simulink model "MsgEthernetMdl"  (R2022a)
settings: Solver=VariableStepAuto  StartTime=0.0  StopTime=30  FixedStep=1  MaxStep=Inf  RelTol=1e-3  EnableMultiTasking=on
PreLoadFcn:
  | load ethernetTypes.mat;
InitFcn:
  | BitRate = 10e6;
values from neighbouring files (symbols this model uses):
  n = length(stations)    [ethernetHubMask.m]
undefined symbols (not defined in the file or in its folder): gateControl, m, networkselector
libraries: matrix_library x4
(part 1 of 2)
settings Model: Creator=The MathWorks, Inc.  LastModifiedBy=lch
settings SolverCC: AlgebraicLoopSolver=TrustRegion
settings DataIOCC: ReturnWorkspaceOutputs=off
settings OptimizationCC: LifeSpan=inf
settings DebuggingCC: UnconnectedInputMsg=warning  UnconnectedOutputMsg=warning  UnconnectedLineMsg=warning  SFUnexpectedBacktrackingDiag=warning  SFNoUnconditionalDefaultTransitionDiag=warning  SFMachineParentedDataDiag=warning  ArithmeticOperatorsInVariantConditions=warning
settings SFSimCC: SimUseLocalCustomCode=off  CustomCodeUndefinedFunction=UseInterfaceOnly
settings RTWCC: RTWUseLocalCustomCode=off
settings CodeAppCC: StateflowObjectComments=on
settings GRTTargetCC: TargetLangStandard=C89/C90 (ANSI)
settings ConfigComp: CovMetricSettings=dw  CovSaveCumulativeToWorkspaceVar=on  CovSaveSingleToWorkspaceVar=on  CovExternalEMLEnable=off

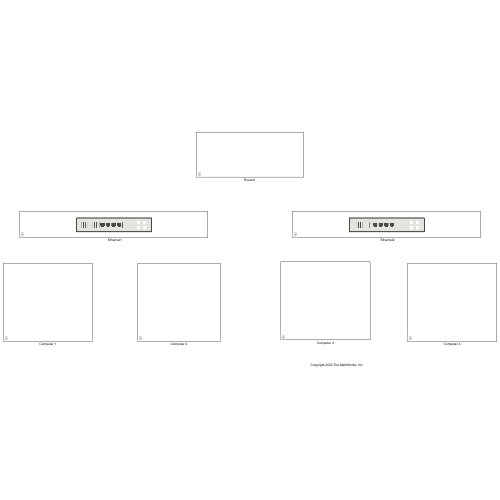
[thumbnail: Simulink's stored preview of the top-level diagram]
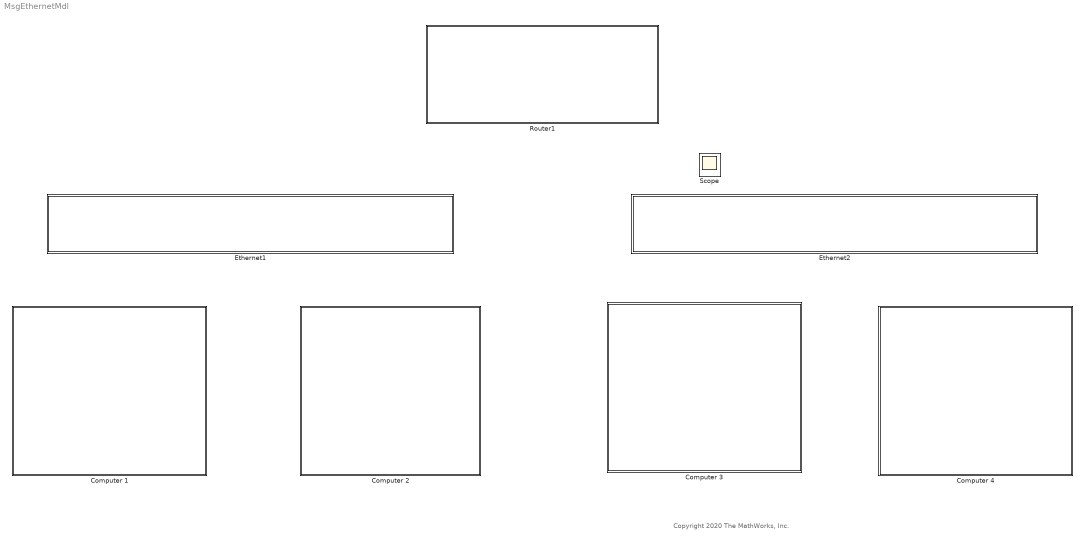
== system MsgEthernetMdl ==
  note: Copyright 2020 The MathWorks, Inc.
  "   Ethernet1" : Subsystem  mask(Ethernet Hub){Stations=[2 1], CableLength=[300 100], PER=[0 0], ProcessingTime=0, ip=[10 1 1 1]}
      mask prompts: Stations "Connected stations"; CableLength "Length of cables (m)"; PER "Packet error rate (PER)"; ProcessingTime "Processing time (s)"
      mask help: Connect Ethernet stations
      mask init:
      | if length(Stations) < 2
      |     error('Number of connected stations must be greater than 1');
      | end
      | if length(CableLength) ~= length(Stations)
      |     error('Parameter ''Length of cables'' must be a vector with number of elements equals to number of connected stations');
      | end
      | if length(PER) ~= length(Stations)
      |     error('Parameter ''Packet error rate'' must be a vector with number of elements equals to number of connected stations');
      | end
      mask DialogControl Container2 Prompt: Parameters
      mask Display: image('ethernet-illustration.png')
  "   Ethernet2" : Subsystem  mask(Ethernet Hub){Stations=[3 2 1], CableLength=[200 300 100], PER=[0 0 0], ProcessingTime=0, ip=[10 1 2 1]}
      mask prompts: Stations "Connected stations"; CableLength "Length of cables (m)"; PER "Packet error rate (PER)"; ProcessingTime "Processing time (s)"
      mask help: Connect Ethernet stations
      mask init: same as MsgEthernetMdl/   Ethernet1
      mask DialogControl Container2 Prompt: Parameters
      mask Display: image('ethernet-illustration.png')
  Computer 1 : Subsystem  mask{ip=[10 1 1 2], netmask=[255 255 255 0], gateway=[10 1 1 1]}
      mask prompts: ip "IP Address"
      mask DialogControl ParameterGroupVar Prompt: 파라미터
  Computer 2 : Subsystem  mask{ip=[10 1 1 3], netmask=[255 255 255 0], gateway=[10 1 1 1]}
      mask prompts: ip "IP Address"
      mask DialogControl ParameterGroupVar Prompt: 파라미터
  Computer 3 : Subsystem  mask{ip=[10 1 2 2], netmask=[255 255 255 0], gateway=[10 1 2 1]}
      mask prompts: ip "IP Address"
      mask DialogControl ParameterGroupVar Prompt: 파라미터
  Computer 4 : Subsystem  mask{ip=[10 1 2 3], netmask=[255 255 255 0], gateway=[10 1 2 1]}
      mask prompts: ip "IP Address"
      mask DialogControl ParameterGroupVar Prompt: 파라미터
  Router1 : Subsystem  mask{vlan1=[10 1 1], vlan2=[10 1 2]}
      mask DialogControl ParameterGroupVar Prompt: 파라미터
  Scope : Scope

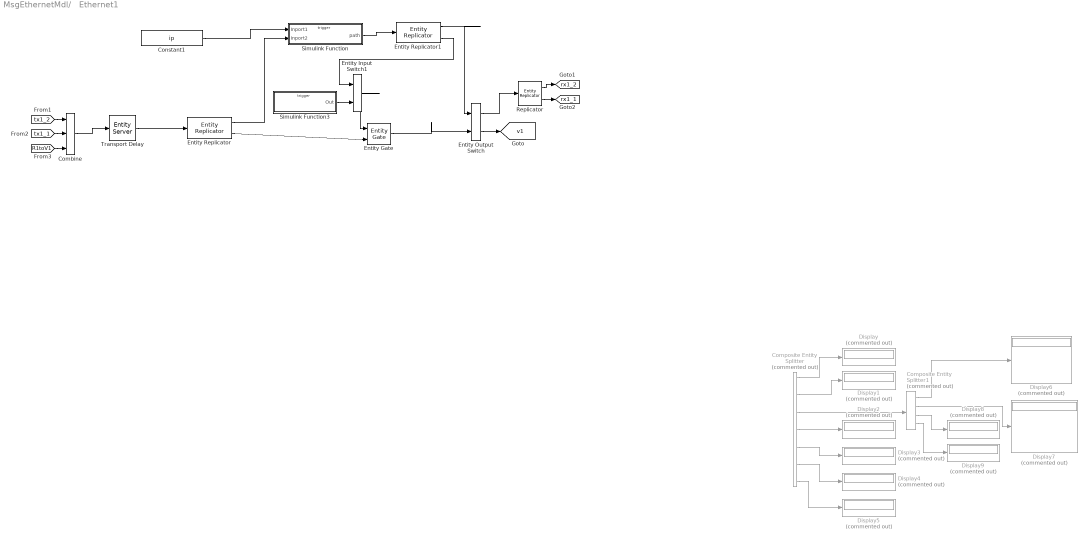
== system MsgEthernetMdl/   Ethernet1 ==
  Combine : EntityInputSwitch  InputPortMessageModes=m,m,m  OutputPortMessageModes=m  NumberInputPorts=3
      settings: InputPortMap=u1,u2,u3
  Composite Entity Splitter : CompositeEntitySplitter  Commented=on  InputPortMessageModes=m  OutputPortMessageModes=m,m,m,m,m,m,m  NumberOutputPorts=7
      settings: OutputPortMap=o0,o1,o2,o3,o4,o5,o6
  Composite Entity Splitter1 : CompositeEntitySplitter  Commented=on  InputPortMessageModes=m  OutputPortMessageModes=m,m,m,m  NumberOutputPorts=4
      settings: OutputPortMap=o0,o1,o2,o3
  Constant1 : Constant  Value=ip
  Display{,1..9} (10 alike) : Display  Commented=on
  Entity Input Switch1 : EntityInputSwitch  InputPortMessageModes=m,m  OutputPortMessageModes=m
  Entity Output Switch : EntityOutputSwitch  InputPortMessageModes=m,m  OutputPortMessageModes=m,m  SwitchingCriterion=From control port  SwitchAttributeName=Attribute1
      settings: InputPortMap=u0,u1
  Entity Gate : EntityGate  InputPortMessageModes=m,m  OutputPortMessageModes=m  OpenGateAtSimulationStart=on
  Entity Replicator : EntityReplicator  InputPortMessageModes=m  OutputPortMessageModes=m,m
  Entity Replicator1 : EntityReplicator  InputPortMessageModes=m  OutputPortMessageModes=m,m
  Replicator : EntityReplicator  InputPortMessageModes=m  OutputPortMessageModes=m,m
  Simulink Function : Subsystem  TreatAsAtomicUnit=on
  Simulink Function3 : Subsystem  TreatAsAtomicUnit=on
  Transport Delay : EntityServer  InputPortMessageModes=m  OutputPortMessageModes=m  Capacity=Inf  ServiceTimeSource=MATLAB action  ServiceTimeAction=|  ServiceCompleteAction=|  ExitAction=gateControl();
      ServiceTimeAction=|
      | src = entity.TxAddress;
      | dst = entity.RxAddress;
      | srcl = 0;
      | dstl = 0;
      | for i = 1:length(Stations)
      |     if src == Stations(i)
      |         srcl = CableLength(i);
      |     end
      |     if dst == Stations(i)
      |         dstl = CableLength(i);
      |     end
      |     if srcl > 0 && dstl > 0
      |         break;
      |     end
      | end
      | dt = ProcessingTime + (srcl + dstl)/3e8;
      ServiceCompleteAction=|
      | networkselector();
      | src = entity.TxAddress;
      | dst = entity.RxAddress;
      | srcIdx = 0;
      | dstIdx = 0;
      | for i = 1:length(Stations)
      |     if src == Stations(i)
      |         srcIdx = i;
      |     end
      |     if dst == Stations(i)
      |         dstIdx = i;
      |     end
      |     if srcIdx > 0 && dstIdx > 0
      |         break;
      |     end
      | end
      | if rand < (PER(srcIdx) + PER(dstIdx))
      |     entity.CRC = 1;
      | end
  tag scope: rx1_1=global, rx1_2=global, v1=global
  wires:
  Combine/1 -> Transport Delay/1
  Transport Delay/1 -> Entity Replicator/1
  [tx1_2] -> Combine/1
  Replicator/1 -> [rx1_2]
  [tx1_1] -> Combine/2
  Replicator/2 -> [rx1_1]
  Entity Output Switch/1 -> Replicator/1
  [R1toV1] -> Combine/3
  Entity Gate/1 -> Entity Output Switch/2
  Simulink Function/1(path) -> Entity Replicator1/1
  Simulink Function3/1(Out) -> Entity Input Switch1/2
  Entity Input Switch1/1 -> Entity Gate/1
  Entity Replicator1/2 -> Entity Input Switch1/1
  Entity Replicator1/1 -> Entity Output Switch/1
  Entity Replicator/2 -> Entity Gate/2
  Entity Replicator/1 -> Simulink Function/2(Inport2)
  Constant1/1 -> Simulink Function/1(Inport1)
  Composite Entity Splitter/2 -> Display1/1
  Composite Entity Splitter1/4 -> Display9/1
  Composite Entity Splitter1/3 -> Display8/1
  Composite Entity Splitter/5 -> Display3/1
  Composite Entity Splitter/4 -> Display2/1
  Composite Entity Splitter/1 -> Display/1
  Composite Entity Splitter/7 -> Display5/1
  Composite Entity Splitter/6 -> Display4/1
  Composite Entity Splitter1/2 -> Display7/1
  Composite Entity Splitter/3 -> Composite Entity Splitter1/1
  Composite Entity Splitter1/1 -> Display6/1
  Entity Output Switch/2 -> [v1]

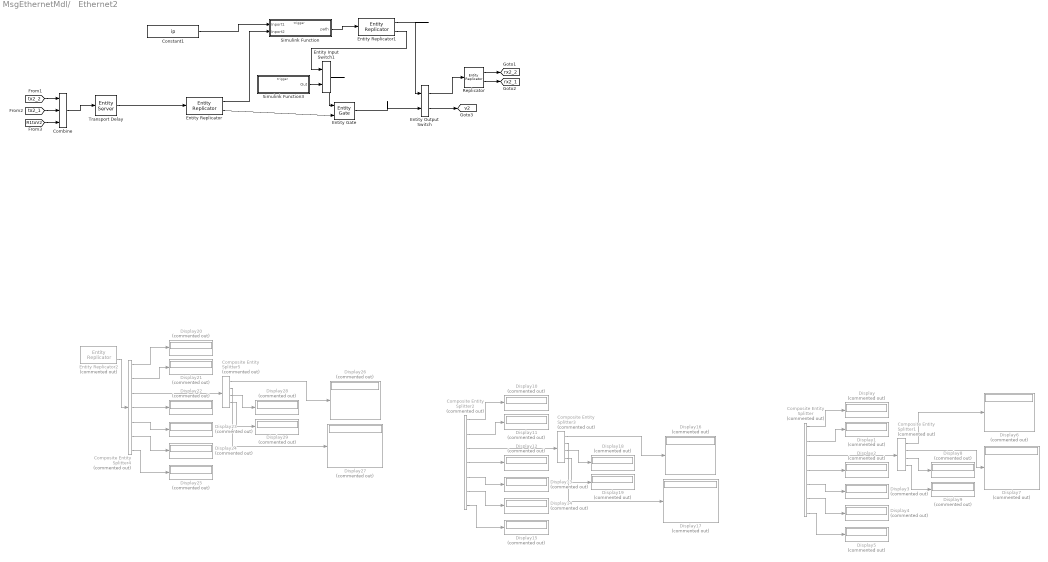
== system MsgEthernetMdl/   Ethernet2 ==
  Combine : EntityInputSwitch  InputPortMessageModes=m,m,m  OutputPortMessageModes=m  NumberInputPorts=3
      settings: InputPortMap=u1,u2,u3
  Composite Entity Splitter : CompositeEntitySplitter  Commented=on  InputPortMessageModes=m  OutputPortMessageModes=m,m,m,m,m,m,m  NumberOutputPorts=7
      settings: OutputPortMap=o0,o1,o2,o3,o4,o5,o6
  Composite Entity Splitter1 : CompositeEntitySplitter  Commented=on  InputPortMessageModes=m  OutputPortMessageModes=m,m,m,m  NumberOutputPorts=4
      settings: OutputPortMap=o0,o1,o2,o3
  Composite Entity Splitter2 : CompositeEntitySplitter  Commented=on  InputPortMessageModes=m  OutputPortMessageModes=m,m,m,m,m,m,m  NumberOutputPorts=7
      settings: OutputPortMap=o0,o1,o2,o3,o4,o5,o6
  Composite Entity Splitter3 : CompositeEntitySplitter  Commented=on  InputPortMessageModes=m  OutputPortMessageModes=m,m,m,m  NumberOutputPorts=4
      settings: OutputPortMap=o0,o1,o2,o3
  Composite Entity Splitter4 : CompositeEntitySplitter  Commented=on  InputPortMessageModes=m  OutputPortMessageModes=m,m,m,m,m,m,m  NumberOutputPorts=7
      settings: OutputPortMap=o0,o1,o2,o3,o4,o5,o6
  Composite Entity Splitter5 : CompositeEntitySplitter  Commented=on  InputPortMessageModes=m  OutputPortMessageModes=m,m,m,m  NumberOutputPorts=4
      settings: OutputPortMap=o0,o1,o2,o3
  Constant1 : Constant  Value=ip
  Display{,1..29} (30 alike) : Display  Commented=on
  Entity Input Switch1 : EntityInputSwitch  InputPortMessageModes=m,m  OutputPortMessageModes=m
  Entity Output Switch : EntityOutputSwitch  InputPortMessageModes=m,m  OutputPortMessageModes=m,m  SwitchingCriterion=From control port  SwitchAttributeName=Attribute1
      settings: InputPortMap=u0,u1
  Entity Gate : EntityGate  InputPortMessageModes=m,m  OutputPortMessageModes=m  OpenGateAtSimulationStart=on
  Entity Replicator : EntityReplicator  InputPortMessageModes=m  OutputPortMessageModes=m,m
  Entity Replicator1 : EntityReplicator  InputPortMessageModes=m  OutputPortMessageModes=m,m
  Entity Replicator2 : EntityReplicator  Commented=on  InputPortMessageModes=m  OutputPortMessageModes=m,m
  Replicator : EntityReplicator  InputPortMessageModes=m  OutputPortMessageModes=m,m
  Simulink Function : Subsystem  TreatAsAtomicUnit=on
  Simulink Function3 : Subsystem  TreatAsAtomicUnit=on
  Transport Delay : EntityServer  InputPortMessageModes=m  OutputPortMessageModes=m  Capacity=Inf  ServiceTimeSource=MATLAB action  ServiceTimeAction=|  ServiceCompleteAction=|  ExitAction=gateControl();
      ServiceTimeAction=|
      | src = entity.TxAddress;
      | dst = entity.RxAddress;
      | srcl = 0;
      | dstl = 0;
      | for i = 1:length(Stations)
      |     if src == Stations(i)
      |         srcl = CableLength(i);
      |     end
      |     if dst == Stations(i)
      |         dstl = CableLength(i);
      |     end
      |     if srcl > 0 && dstl > 0
      |         break;
      |     end
      | end
      | dt = ProcessingTime + (srcl + dstl)/3e8;
      ServiceCompleteAction=|
      | networkselector();
      | src = entity.TxAddress;
      | dst = entity.RxAddress;
      | srcIdx = 0;
      | dstIdx = 0;
      | for i = 1:length(Stations)
      |     if src == Stations(i)
      |         srcIdx = i;
      |     end
      |     if dst == Stations(i)
      |         dstIdx = i;
      |     end
      |     if srcIdx > 0 && dstIdx > 0
      |         break;
      |     end
      | end
      | if rand < (PER(srcIdx) + PER(dstIdx))
      |     entity.CRC = 1;
      | end
  tag scope: rx2_1=global, rx2_2=global, v2=global
  wires:
  Combine/1 -> Transport Delay/1
  Entity Output Switch/1 -> Replicator/1
  [tx2_2] -> Combine/1
  Replicator/1 -> [rx2_2]
  [tx2_1] -> Combine/2
  Replicator/2 -> [rx2_1]
  [R1toV2] -> Combine/3
  Composite Entity Splitter1/2 -> Display7/1
  Composite Entity Splitter1/4 -> Display9/1
  Composite Entity Splitter/7 -> Display5/1
  Composite Entity Splitter/1 -> Display/1
  Composite Entity Splitter/2 -> Display1/1
  Composite Entity Splitter/6 -> Display4/1
  Composite Entity Splitter/4 -> Display2/1
  Composite Entity Splitter1/3 -> Display8/1
  Composite Entity Splitter/3 -> Composite Entity Splitter1/1
  Composite Entity Splitter1/1 -> Display6/1
  Composite Entity Splitter/5 -> Display3/1
  Composite Entity Splitter2/5 -> Display13/1
  Composite Entity Splitter3/1 -> Display16/1
  Composite Entity Splitter2/3 -> Composite Entity Splitter3/1
  Composite Entity Splitter3/3 -> Display18/1
  Composite Entity Splitter2/4 -> Display12/1
  Composite Entity Splitter2/6 -> Display14/1
  Composite Entity Splitter2/2 -> Display11/1
  Composite Entity Splitter2/1 -> Display10/1
  Composite Entity Splitter2/7 -> Display15/1
  Composite Entity Splitter3/4 -> Display19/1
  Composite Entity Splitter3/2 -> Display17/1
  Entity Replicator/1 -> Simulink Function/2(Inport2)
  Constant1/1 -> Simulink Function/1(Inport1)
  Entity Replicator1/1 -> Entity Output Switch/1
  Entity Replicator1/2 -> Entity Input Switch1/1
  Entity Input Switch1/1 -> Entity Gate/1
  Simulink Function/1(path) -> Entity Replicator1/1
  Simulink Function3/1(Out) -> Entity Input Switch1/2
  Entity Gate/1 -> Entity Output Switch/2
  Entity Replicator/2 -> Entity Gate/2
  Transport Delay/1 -> Entity Replicator/1
  Composite Entity Splitter5/1 -> Display26/1
  Composite Entity Splitter4/7 -> Display25/1
  Composite Entity Splitter4/5 -> Display23/1
  Composite Entity Splitter5/2 -> Display27/1
  Composite Entity Splitter4/6 -> Display24/1
  Composite Entity Splitter4/2 -> Display21/1
  Composite Entity Splitter5/3 -> Display28/1
  Composite Entity Splitter4/1 -> Display20/1
  Composite Entity Splitter5/4 -> Display29/1
  Composite Entity Splitter4/3 -> Composite Entity Splitter5/1
  Composite Entity Splitter4/4 -> Display22/1
  Entity Replicator2/2 -> Composite Entity Splitter4/1
  Entity Output Switch/2 -> [v2]

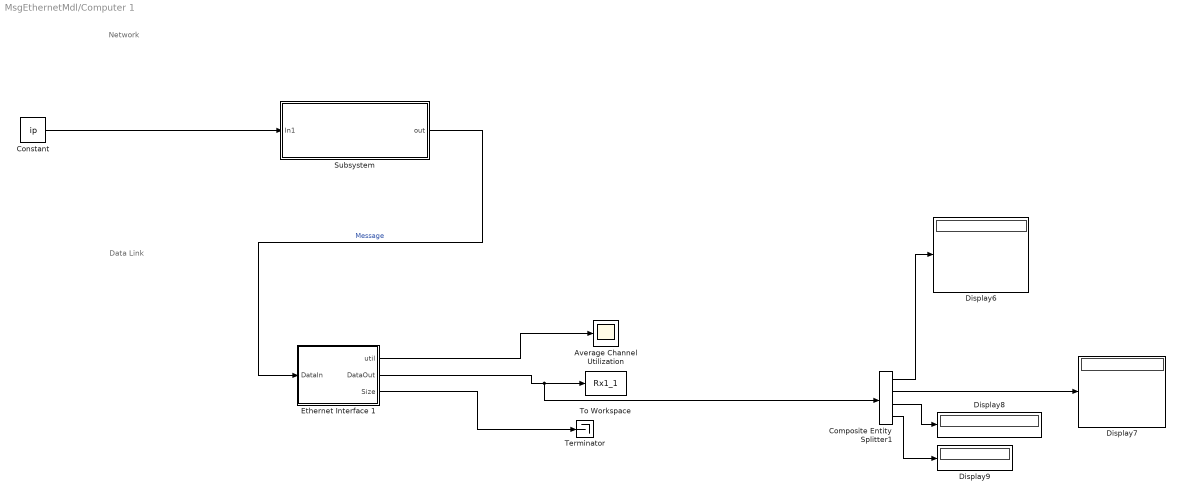
== system MsgEthernetMdl/Computer 1 ==
  note: Network
  note: Data Link
  Average Channel Utilization : Scope
  Composite Entity Splitter1 : CompositeEntitySplitter  InputPortMessageModes=m  OutputPortMessageModes=m,m,m,m  NumberOutputPorts=4
      settings: OutputPortMap=o0,o1,o2,o3
  Constant : Constant  Value=ip
  Display{6..9} (4 alike) : Display
  Ethernet Interface 1 : Subsystem  mask(Ethernet MAC Layer){StationID=1, TxBufferCapacity=256}
      mask prompts: StationID "Station ID"; TxBufferCapacity "Transmission buffer capacity"
      mask help: Ethernet MAC layer packet transmission and reception based on CSMA/CD
      mask Display: image('ethernet-interface-illustration.png')
  Subsystem : Subsystem
  Terminator : Terminator
  To Workspace : ToWorkspace  VariableName=Rx1_1  SaveFormat=Timeseries  SampleTime=-1
  wires:
  Ethernet Interface 1/3(Size) -> Terminator/1
  Subsystem/1(out) -> Ethernet Interface 1/1(DataIn)  "Message"
  Ethernet Interface 1/1(util) -> Average Channel Utilization/1
  Constant/1 -> Subsystem/1(In1)
  Composite Entity Splitter1/1 -> Display6/1
  Composite Entity Splitter1/3 -> Display8/1
  Composite Entity Splitter1/4 -> Display9/1
  Composite Entity Splitter1/2 -> Display7/1
  Ethernet Interface 1/2(DataOut) -> Composite Entity Splitter1/1, To Workspace/1

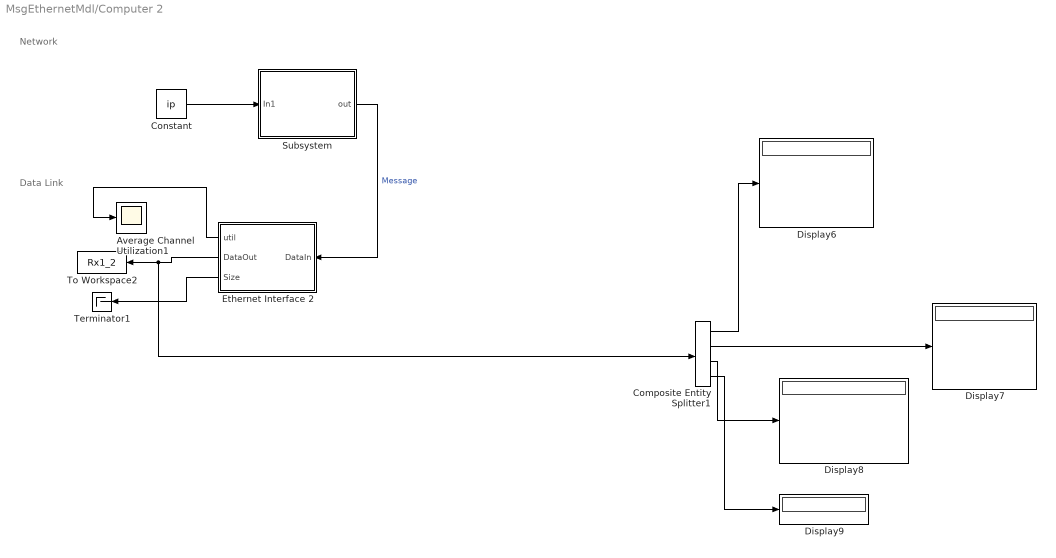
== system MsgEthernetMdl/Computer 2 ==
  note: Network
  note: Data Link
  Average Channel Utilization1 : Scope
  Composite Entity Splitter1 : CompositeEntitySplitter  InputPortMessageModes=m  OutputPortMessageModes=m,m,m,m  NumberOutputPorts=4
      settings: OutputPortMap=o0,o1,o2,o3
  Constant : Constant  Value=ip
  Display{6..9} (4 alike) : Display
  Ethernet Interface 2 : Subsystem  mask(Ethernet MAC Layer){StationID=2, TxBufferCapacity=256}
      mask prompts: StationID "Station ID"; TxBufferCapacity "Transmission buffer capacity"
      mask help: Ethernet MAC layer packet transmission and reception based on CSMA/CD
      mask Display: image('ethernet-interface-illustration.png')
  Subsystem : Subsystem
  Terminator1 : Terminator
  To Workspace2 : ToWorkspace  VariableName=Rx1_2  SaveFormat=Timeseries  SampleTime=-1
  wires:
  Ethernet Interface 2/3(Size) -> Terminator1/1
  Subsystem/1(out) -> Ethernet Interface 2/1(DataIn)  "Message"
  Ethernet Interface 2/1(util) -> Average Channel Utilization1/1
  Constant/1 -> Subsystem/1(In1)
  Composite Entity Splitter1/3 -> Display8/1
  Composite Entity Splitter1/2 -> Display7/1
  Composite Entity Splitter1/4 -> Display9/1
  Composite Entity Splitter1/1 -> Display6/1
  Ethernet Interface 2/2(DataOut) -> Composite Entity Splitter1/1, To Workspace2/1

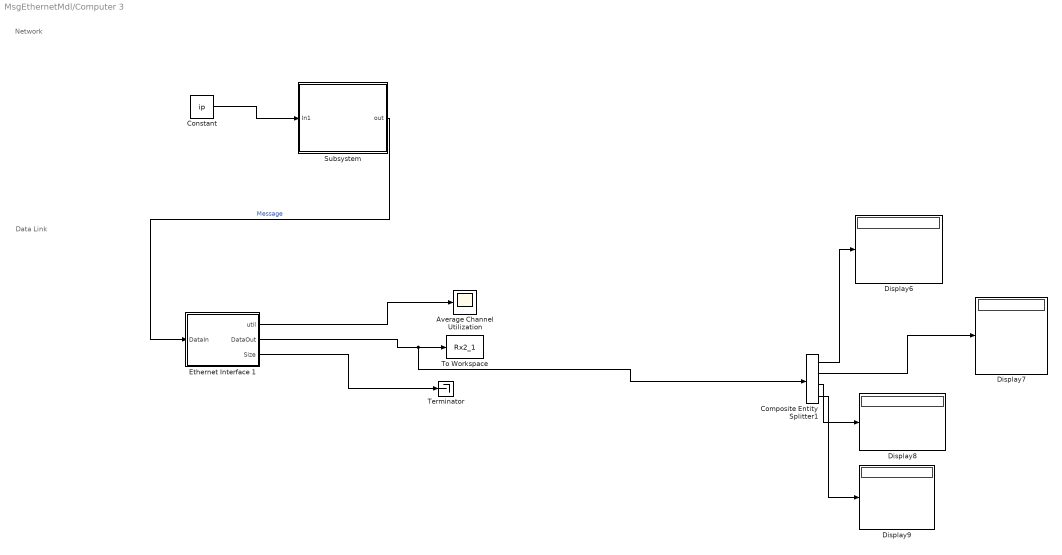
== system MsgEthernetMdl/Computer 3 ==
  note: Network
  note: Data Link
  Average Channel Utilization : Scope
  Composite Entity Splitter1 : CompositeEntitySplitter  InputPortMessageModes=m  OutputPortMessageModes=m,m,m,m  NumberOutputPorts=4
      settings: OutputPortMap=o0,o1,o2,o3
  Constant : Constant  Value=ip
  Display{6..9} (4 alike) : Display
  Ethernet Interface 1 : Subsystem  mask(Ethernet MAC Layer){StationID=1, TxBufferCapacity=256}
      mask prompts: StationID "Station ID"; TxBufferCapacity "Transmission buffer capacity"
      mask help: Ethernet MAC layer packet transmission and reception based on CSMA/CD
      mask Display: image('ethernet-interface-illustration.png')
  Subsystem : Subsystem
  Terminator : Terminator
  To Workspace : ToWorkspace  VariableName=Rx2_1  SaveFormat=Timeseries  SampleTime=-1
  wires:
  Ethernet Interface 1/3(Size) -> Terminator/1
  Subsystem/1(out) -> Ethernet Interface 1/1(DataIn)  "Message"
  Ethernet Interface 1/1(util) -> Average Channel Utilization/1
  Constant/1 -> Subsystem/1(In1)
  Ethernet Interface 1/2(DataOut) -> Composite Entity Splitter1/1, To Workspace/1
  Composite Entity Splitter1/3 -> Display8/1
  Composite Entity Splitter1/2 -> Display7/1
  Composite Entity Splitter1/4 -> Display9/1
  Composite Entity Splitter1/1 -> Display6/1

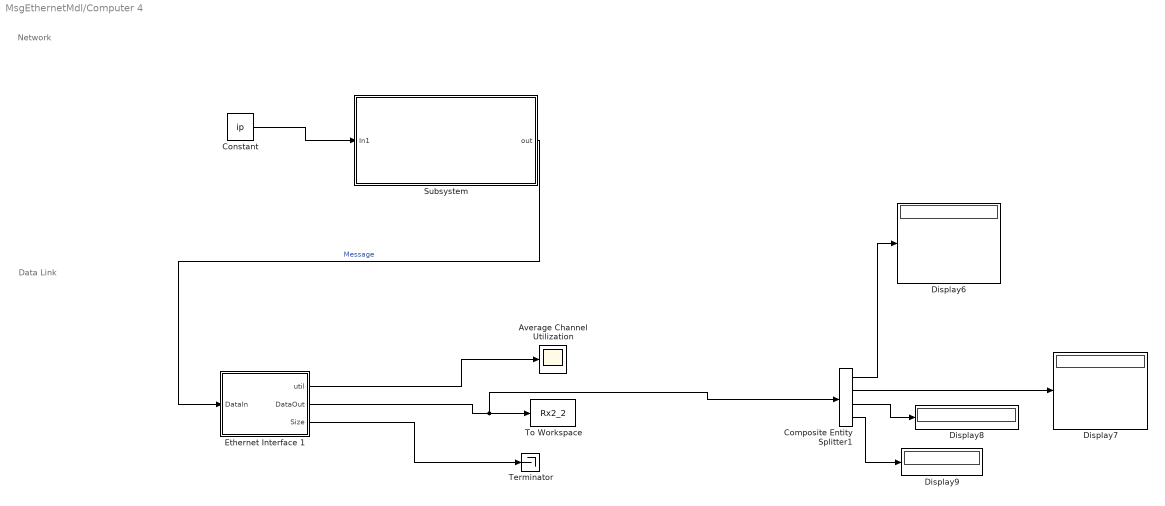
== system MsgEthernetMdl/Computer 4 ==
  note: Network
  note: Data Link
  Average Channel Utilization : Scope
  Composite Entity Splitter1 : CompositeEntitySplitter  InputPortMessageModes=m  OutputPortMessageModes=m,m,m,m  NumberOutputPorts=4
      settings: OutputPortMap=o0,o1,o2,o3
  Constant : Constant  Value=ip
  Display{6..9} (4 alike) : Display
  Ethernet Interface 1 : Subsystem  mask(Ethernet MAC Layer){StationID=2, TxBufferCapacity=256}
      mask prompts: StationID "Station ID"; TxBufferCapacity "Transmission buffer capacity"
      mask help: Ethernet MAC layer packet transmission and reception based on CSMA/CD
      mask Display: image('ethernet-interface-illustration.png')
  Subsystem : Subsystem
  Terminator : Terminator
  To Workspace : ToWorkspace  VariableName=Rx2_2  SaveFormat=Timeseries  SampleTime=-1
  wires:
  Ethernet Interface 1/3(Size) -> Terminator/1
  Subsystem/1(out) -> Ethernet Interface 1/1(DataIn)  "Message"
  Ethernet Interface 1/1(util) -> Average Channel Utilization/1
  Constant/1 -> Subsystem/1(In1)
  Composite Entity Splitter1/3 -> Display8/1
  Composite Entity Splitter1/1 -> Display6/1
  Composite Entity Splitter1/4 -> Display9/1
  Composite Entity Splitter1/2 -> Display7/1
  Ethernet Interface 1/2(DataOut) -> Composite Entity Splitter1/1, To Workspace/1

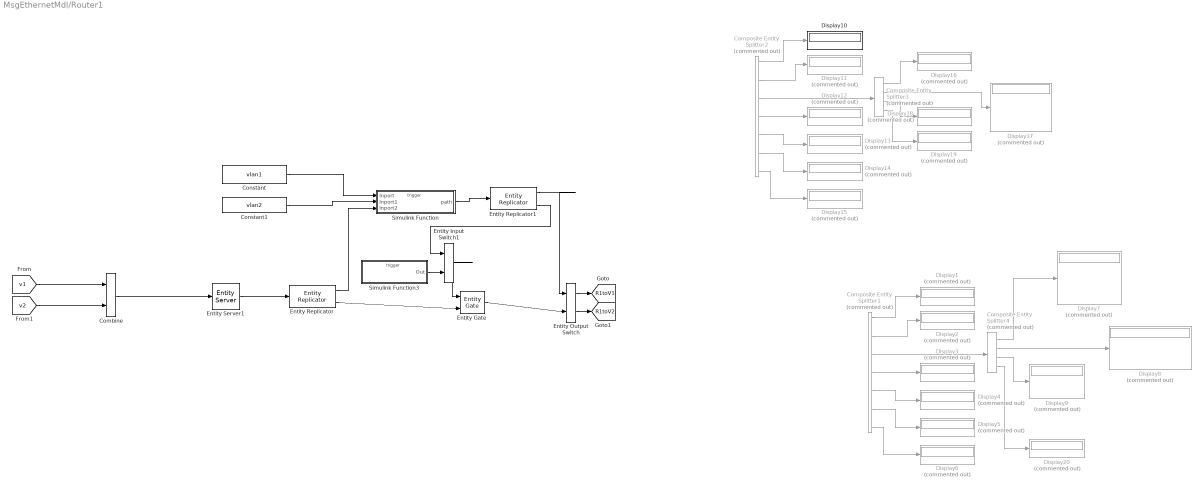
== system MsgEthernetMdl/Router1 ==
  Combine : EntityInputSwitch  InputPortMessageModes=m,m  OutputPortMessageModes=m
  Composite Entity Splitter1 : CompositeEntitySplitter  Commented=on  InputPortMessageModes=m  OutputPortMessageModes=m,m,m,m,m,m,m  NumberOutputPorts=7
      settings: OutputPortMap=o0,o1,o2,o3,o4,o5,o6
  Composite Entity Splitter2 : CompositeEntitySplitter  Commented=on  InputPortMessageModes=m  OutputPortMessageModes=m,m,m,m,m,m,m  NumberOutputPorts=7
      settings: OutputPortMap=o0,o1,o2,o3,o4,o5,o6
  Composite Entity Splitter3 : CompositeEntitySplitter  Commented=on  InputPortMessageModes=m  OutputPortMessageModes=m,m,m,m  NumberOutputPorts=4
      settings: OutputPortMap=o0,o1,o2,o3
  Composite Entity Splitter4 : CompositeEntitySplitter  Commented=on  InputPortMessageModes=m  OutputPortMessageModes=m,m,m,m  NumberOutputPorts=4
      settings: OutputPortMap=o0,o1,o2,o3
  Constant : Constant  Value=vlan1
  Constant1 : Constant  Value=vlan2
  Display{1..9,11..20} (19 alike) : Display  Commented=on
  Display10 : Display
  Entity Input Switch1 : EntityInputSwitch  InputPortMessageModes=m,m  OutputPortMessageModes=m
  Entity Output Switch : EntityOutputSwitch  InputPortMessageModes=m,m  OutputPortMessageModes=m,m  SwitchingCriterion=From control port  SwitchAttributeName=Attribute1
      settings: InputPortMap=u0,u1
  Entity Gate : EntityGate  InputPortMessageModes=m,m  OutputPortMessageModes=m  OpenGateAtSimulationStart=on
  Entity Replicator : EntityReplicator  InputPortMessageModes=m  OutputPortMessageModes=m,m
  Entity Replicator1 : EntityReplicator  InputPortMessageModes=m  OutputPortMessageModes=m,m
  Entity Server1 : EntityServer  InputPortMessageModes=m  OutputPortMessageModes=m  Capacity=inf  ServiceTimeSource=MATLAB action  ServiceCompleteAction=networkselector();  ExitAction=gateControl();
  Simulink Function : Subsystem  TreatAsAtomicUnit=on
  Simulink Function3 : Subsystem  TreatAsAtomicUnit=on
  tag scope: R1toV1=global, R1toV2=global
  wires:
  [v1] -> Combine/1
  Composite Entity Splitter3/4 -> Display19/1
  Composite Entity Splitter2/3 -> Composite Entity Splitter3/1
  Composite Entity Splitter2/5 -> Display13/1
  Composite Entity Splitter2/6 -> Display14/1
  Composite Entity Splitter2/2 -> Display11/1
  Composite Entity Splitter2/7 -> Display15/1
  Composite Entity Splitter3/1 -> Display16/1
  Composite Entity Splitter3/2 -> Display17/1
  Composite Entity Splitter3/3 -> Display18/1
  Composite Entity Splitter2/1 -> Display10/1
  Composite Entity Splitter2/4 -> Display12/1
  Composite Entity Splitter1/1 -> Display1/1
  Composite Entity Splitter4/3 -> Display9/1
  Composite Entity Splitter4/1 -> Display7/1
  Composite Entity Splitter1/5 -> Display4/1
  Composite Entity Splitter1/3 -> Composite Entity Splitter4/1
  Composite Entity Splitter1/4 -> Display3/1
  Composite Entity Splitter4/2 -> Display8/1
  Composite Entity Splitter1/7 -> Display6/1
  Composite Entity Splitter1/2 -> Display2/1
  Composite Entity Splitter4/4 -> Display20/1
  Composite Entity Splitter1/6 -> Display5/1
  [v2] -> Combine/2
  Combine/1 -> Entity Server1/1
  Entity Replicator/2 -> Entity Gate/2
  Entity Gate/1 -> Entity Output Switch/2
  Simulink Function/1(path) -> Entity Replicator1/1
  Entity Input Switch1/1 -> Entity Gate/1
  Simulink Function3/1(Out) -> Entity Input Switch1/2
  Entity Replicator1/2 -> Entity Input Switch1/1
  Entity Replicator1/1 -> Entity Output Switch/1
  Constant1/1 -> Simulink Function/2(Inport1)
  Constant/1 -> Simulink Function/1(Inport)
  Entity Server1/1 -> Entity Replicator/1
  Entity Replicator/1 -> Simulink Function/3(Inport2)
  Entity Output Switch/2 -> [R1toV2]
  Entity Output Switch/1 -> [R1toV1]

== system MsgEthernetMdl/   Ethernet1/Simulink Function ==
  Inport1 : Inport
  Inport2 : Inport  Port=2
  networkselector : TriggerPort  TriggerType=function-call  IsSimulinkFunction=on  FunctionName=networkselector  FunctionVisibility=scoped  VariantControl=(inherit)
  Bus Selector : BusSelector  OutputSignals=Data
  Bus Selector1 : BusSelector  OutputSignals=DestAddress
  Display : Display
  MATLAB Function : MATLAB Function  TreatAsAtomicUnit=on
  Message Send : Send  OutputPortMessageModes=m
  Receive : Receive  InputPortMessageModes=m  UseInternalQueue=off  QueueOverwriting=on  QueueLength=1  QueueType=LIFO
  path : Outport
  wires:
  Receive/1 -> Bus Selector/1
  Inport1/1 -> MATLAB Function/1(v1)
  Bus Selector/1 -> Bus Selector1/1  "<Data>"
  MATLAB Function/1(idx) -> Display/1, Message Send/1
  Message Send/1 -> path/1
  Inport2/1 -> Receive/1
  Bus Selector1/1 -> MATLAB Function/2(dest)  "<DestAddress>"

== system MsgEthernetMdl/   Ethernet1/Simulink Function3 ==
  gateControl : TriggerPort  TriggerType=function-call  IsSimulinkFunction=on  FunctionName=gateControl  FunctionVisibility=scoped  VariantControl=Variant
  Constant : Constant  Value=0
  Message Send : Send  OutputPortMessageModes=m
  Out : Outport
  wires:
  Message Send/1 -> Out/1
  Constant/1 -> Message Send/1

== system MsgEthernetMdl/   Ethernet2/Simulink Function ==
  Inport1 : Inport
  Inport2 : Inport  Port=2
  networkselector : TriggerPort  TriggerType=function-call  IsSimulinkFunction=on  FunctionName=networkselector  FunctionVisibility=scoped  VariantControl=(inherit)
  Bus Selector : BusSelector  OutputSignals=Data
  Bus Selector1 : BusSelector  OutputSignals=DestAddress
  Display : Display
  MATLAB Function : MATLAB Function  TreatAsAtomicUnit=on
  Message Send : Send  OutputPortMessageModes=m
  Receive : Receive  InputPortMessageModes=m  UseInternalQueue=off  QueueOverwriting=on  QueueLength=1  QueueType=LIFO
  path : Outport
  wires:
  Receive/1 -> Bus Selector/1
  Inport1/1 -> MATLAB Function/1(v1)
  Bus Selector/1 -> Bus Selector1/1  "<Data>"
  MATLAB Function/1(idx) -> Display/1, Message Send/1
  Message Send/1 -> path/1
  Inport2/1 -> Receive/1
  Bus Selector1/1 -> MATLAB Function/2(dest)  "<DestAddress>"

== system MsgEthernetMdl/   Ethernet2/Simulink Function3 ==
  gateControl : TriggerPort  TriggerType=function-call  IsSimulinkFunction=on  FunctionName=gateControl  FunctionVisibility=scoped  VariantControl=Variant
  Constant : Constant  Value=0
  Message Send : Send  OutputPortMessageModes=m
  Out : Outport
  wires:
  Message Send/1 -> Out/1
  Constant/1 -> Message Send/1

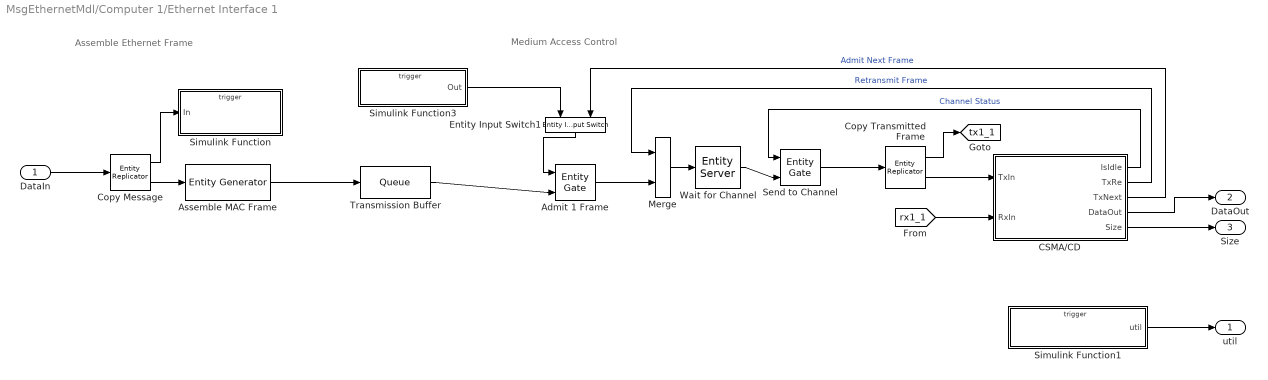
== system MsgEthernetMdl/Computer 1/Ethernet Interface 1 ==
  note: Assemble Ethernet Frame
  note: Medium Access Control
  DataIn : Inport
  "Admit 1 Frame " : EntityGate  InputPortMessageModes=m,m  OutputPortMessageModes=m  OpenGateAtSimulationStart=on
  Assemble MAC Frame : EntityGenerator  InputPortMessageModes=m  OutputPortMessageModes=m  GenerationMethod=Event-based  GenerateAction=|  EntityType=Bus object  EntityTypeName=ethernetPacket
      | entity.TxAddress = StationID;
      | [entity.Data, entity.RxAddress, entity.PayloadSize] = initPacket();
      | entity.TxDelay = (entity.PayloadSize+22)*8/BitRate;
      | entity.BackoffTime = 0;
      | entity.CRC = 0;
      settings: InputPortMap=u0
  CSMA/CD : Stateflow chart  TreatAsAtomicUnit=on
  Copy Message : EntityReplicator  InputPortMessageModes=m  OutputPortMessageModes=m,m
  Copy Transmitted Frame : EntityReplicator  InputPortMessageModes=m  OutputPortMessageModes=m,m
  Entity Input Switch1 : EntityInputSwitch  InputPortMessageModes=m,m  OutputPortMessageModes=m
  "Merge " : EntityInputSwitch  InputPortMessageModes=m,m  OutputPortMessageModes=m
  Send to Channel : EntityGate  InputPortMessageModes=m,m  OutputPortMessageModes=m  OpenGateAtSimulationStart=on
  Simulink Function : Subsystem  TreatAsAtomicUnit=on
  Simulink Function1 : Subsystem  TreatAsAtomicUnit=on
  Simulink Function3 : Subsystem  TreatAsAtomicUnit=on
  Transmission Buffer : Queue  InputPortMessageModes=m  OutputPortMessageModes=m  Capacity=TxBufferCapacity  ExitAction=gateControl();
  Wait for Channel : EntityServer  InputPortMessageModes=m  OutputPortMessageModes=m  Capacity=1  ServiceTimeSource=Attribute  ServiceTimeAttributeName=BackoffTime
  util : Outport
  DataOut : Outport  Port=2
  Size : Outport  Port=3
  tag scope: tx1_1=global
  wires:
  CSMA/CD/5(Size) -> Size/1
  Simulink Function1/1(util) -> util/1
  CSMA/CD/4(DataOut) -> DataOut/1
  CSMA/CD/1(IsIdle) -> Send to Channel/1  "Channel Status"
  CSMA/CD/3(TxNext) -> Entity Input Switch1/2  "Admit Next Frame"
  Transmission Buffer/1 -> "Admit 1 Frame "/2
  "Admit 1 Frame "/1 -> "Merge "/2
  "Merge "/1 -> Wait for Channel/1
  Wait for Channel/1 -> Send to Channel/2
  Send to Channel/1 -> Copy Transmitted Frame/1
  Copy Transmitted Frame/2 -> CSMA/CD/1(TxIn)
  [rx1_1] -> CSMA/CD/2(RxIn)
  CSMA/CD/2(TxRe) -> "Merge "/1  "Retransmit Frame"
  Copy Transmitted Frame/1 -> [tx1_1]
  Assemble MAC Frame/1 -> Transmission Buffer/1
  DataIn/1 -> Copy Message/1
  Copy Message/2 -> Assemble MAC Frame/1
  Copy Message/1 -> Simulink Function/1(In)
  Entity Input Switch1/1 -> "Admit 1 Frame "/1
  Simulink Function3/1(Out) -> Entity Input Switch1/1

== system MsgEthernetMdl/Computer 1/Subsystem ==
  In1 : Inport
  Bus Creator : BusCreator  Inputs=4  OutDataTypeStr=Bus: dataPacket  NonVirtualBus=on
  Constant : Constant  Value=[10 1 2 3]
  Generate Data 1 : MATLAB Function  TreatAsAtomicUnit=on  SystemSampleTime=0.2
  Send : Send  OutputPortMessageModes=m
  out : Outport  InputPortMessageModes=m  OutDataTypeStr=Bus: dataPacket  BusOutputAsStruct=on
  wires:
  Constant/1 -> Bus Creator/2  "DestAddress"
  In1/1 -> Bus Creator/1  "SrcAddress"
  Send/1 -> out/1  "Message"
  Generate Data 1/2(PayloadSize) -> Bus Creator/4
  Bus Creator/1 -> Send/1
  Generate Data 1/1(Data) -> Bus Creator/3

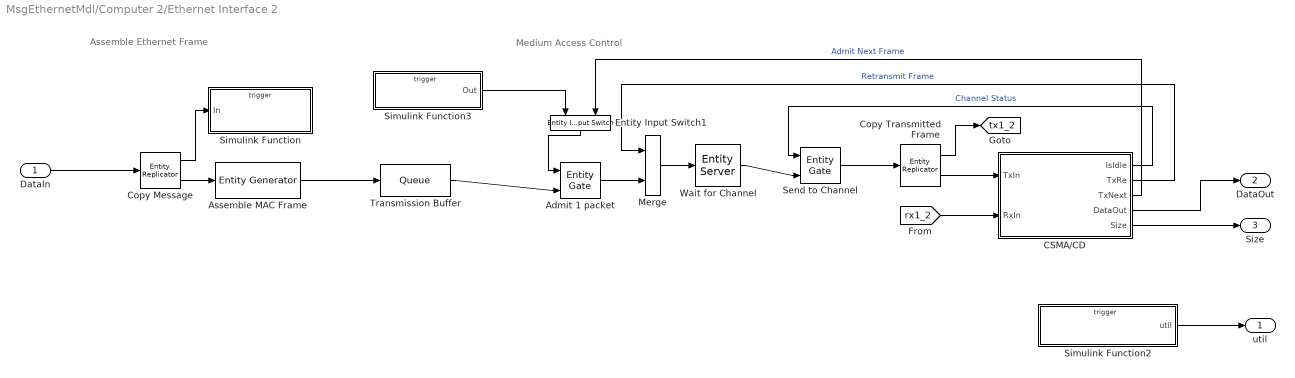
== system MsgEthernetMdl/Computer 2/Ethernet Interface 2 ==
  note: Medium Access Control
  note: Assemble Ethernet Frame
  DataIn : Inport
  "Admit 1 packet " : EntityGate  InputPortMessageModes=m,m  OutputPortMessageModes=m  OpenGateAtSimulationStart=on
  Assemble MAC Frame : EntityGenerator  InputPortMessageModes=m  OutputPortMessageModes=m  GenerationMethod=Event-based  GenerateAction=|  EntityType=Bus object  EntityTypeName=ethernetPacket
      | entity.TxAddress = StationID;
      | [entity.Data, entity.RxAddress, entity.PayloadSize] = initPacket();
      | entity.TxDelay = (entity.PayloadSize+22)*8/BitRate;
      | entity.BackoffTime = 0;
      | entity.CRC = 0;
      settings: InputPortMap=u0
  CSMA/CD : Stateflow chart  TreatAsAtomicUnit=on
  Copy Message : EntityReplicator  InputPortMessageModes=m  OutputPortMessageModes=m,m
  Copy Transmitted Frame : EntityReplicator  InputPortMessageModes=m  OutputPortMessageModes=m,m
  Entity Input Switch1 : EntityInputSwitch  InputPortMessageModes=m,m  OutputPortMessageModes=m
  Merge : EntityInputSwitch  InputPortMessageModes=m,m  OutputPortMessageModes=m
  Send to Channel : EntityGate  InputPortMessageModes=m,m  OutputPortMessageModes=m  OpenGateAtSimulationStart=on
  Simulink Function : Subsystem  TreatAsAtomicUnit=on
  Simulink Function2 : Subsystem  TreatAsAtomicUnit=on
  Simulink Function3 : Subsystem  TreatAsAtomicUnit=on
  Transmission Buffer : Queue  InputPortMessageModes=m  OutputPortMessageModes=m  Capacity=TxBufferCapacity  ExitAction=gateControl();
  Wait for Channel : EntityServer  InputPortMessageModes=m  OutputPortMessageModes=m  Capacity=1  ServiceTimeSource=Attribute  ServiceTimeAttributeName=BackoffTime
  util : Outport
  DataOut : Outport  Port=2
  Size : Outport  Port=3
  tag scope: tx1_2=global
  wires:
  CSMA/CD/5(Size) -> Size/1
  Simulink Function2/1(util) -> util/1
  CSMA/CD/4(DataOut) -> DataOut/1
  CSMA/CD/1(IsIdle) -> Send to Channel/1  "Channel Status"
  CSMA/CD/3(TxNext) -> Entity Input Switch1/2  "Admit Next Frame"
  Transmission Buffer/1 -> "Admit 1 packet "/2
  "Admit 1 packet "/1 -> Merge/2
  Merge/1 -> Wait for Channel/1
  Wait for Channel/1 -> Send to Channel/2
  Send to Channel/1 -> Copy Transmitted Frame/1
  Copy Transmitted Frame/2 -> CSMA/CD/1(TxIn)
  [rx1_2] -> CSMA/CD/2(RxIn)
  CSMA/CD/2(TxRe) -> Merge/1  "Retransmit Frame"
  Copy Transmitted Frame/1 -> [tx1_2]
  Assemble MAC Frame/1 -> Transmission Buffer/1
  DataIn/1 -> Copy Message/1
  Copy Message/2 -> Assemble MAC Frame/1
  Copy Message/1 -> Simulink Function/1(In)
  Simulink Function3/1(Out) -> Entity Input Switch1/1
  Entity Input Switch1/1 -> "Admit 1 packet "/1

== system MsgEthernetMdl/Computer 2/Subsystem ==
  In1 : Inport
  Bus Creator : BusCreator  Inputs=4  OutDataTypeStr=Bus: dataPacket  NonVirtualBus=on
  Constant : Constant  Value=[10 1 2 2]
  Generate Data 1 : MATLAB Function  TreatAsAtomicUnit=on  SystemSampleTime=0.3
  Send : Send  OutputPortMessageModes=m
  out : Outport  InputPortMessageModes=m  OutDataTypeStr=Bus: dataPacket  BusOutputAsStruct=on
  wires:
  Constant/1 -> Bus Creator/2  "DestAddress"
  In1/1 -> Bus Creator/1  "SrcAddress"
  Send/1 -> out/1  "Message"
  Generate Data 1/2(PayloadSize) -> Bus Creator/4
  Bus Creator/1 -> Send/1
  Generate Data 1/1(Data) -> Bus Creator/3

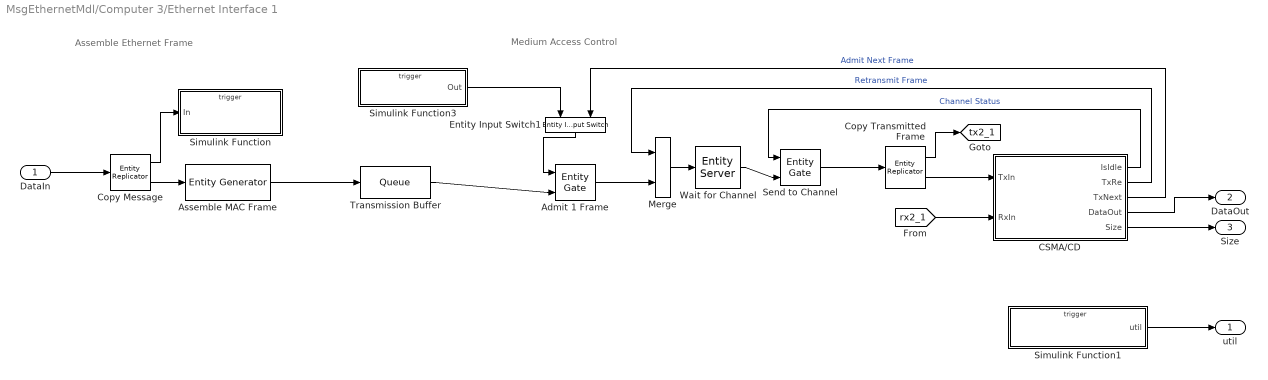
== system MsgEthernetMdl/Computer 3/Ethernet Interface 1 ==
  note: Assemble Ethernet Frame
  note: Medium Access Control
  DataIn : Inport
  "Admit 1 Frame " : EntityGate  InputPortMessageModes=m,m  OutputPortMessageModes=m  OpenGateAtSimulationStart=on
  Assemble MAC Frame : EntityGenerator  InputPortMessageModes=m  OutputPortMessageModes=m  GenerationMethod=Event-based  GenerateAction=|  EntityType=Bus object  EntityTypeName=ethernetPacket
      | entity.TxAddress = StationID;
      | [entity.Data, entity.RxAddress, entity.PayloadSize] = initPacket();
      | entity.TxDelay = (entity.PayloadSize+22)*8/BitRate;
      | entity.BackoffTime = 0;
      | entity.CRC = 0;
      settings: InputPortMap=u0
  CSMA/CD : Stateflow chart  TreatAsAtomicUnit=on
  Copy Message : EntityReplicator  InputPortMessageModes=m  OutputPortMessageModes=m,m
  Copy Transmitted Frame : EntityReplicator  InputPortMessageModes=m  OutputPortMessageModes=m,m
  Entity Input Switch1 : EntityInputSwitch  InputPortMessageModes=m,m  OutputPortMessageModes=m
  "Merge " : EntityInputSwitch  InputPortMessageModes=m,m  OutputPortMessageModes=m
  Send to Channel : EntityGate  InputPortMessageModes=m,m  OutputPortMessageModes=m  OpenGateAtSimulationStart=on
  Simulink Function : Subsystem  TreatAsAtomicUnit=on
  Simulink Function1 : Subsystem  TreatAsAtomicUnit=on
  Simulink Function3 : Subsystem  TreatAsAtomicUnit=on
  Transmission Buffer : Queue  InputPortMessageModes=m  OutputPortMessageModes=m  Capacity=TxBufferCapacity  ExitAction=gateControl();
  Wait for Channel : EntityServer  InputPortMessageModes=m  OutputPortMessageModes=m  Capacity=1  ServiceTimeSource=Attribute  ServiceTimeAttributeName=BackoffTime
  util : Outport
  DataOut : Outport  Port=2
  Size : Outport  Port=3
  tag scope: tx2_1=global
  wires:
  CSMA/CD/5(Size) -> Size/1
  Simulink Function1/1(util) -> util/1
  CSMA/CD/4(DataOut) -> DataOut/1
  CSMA/CD/1(IsIdle) -> Send to Channel/1  "Channel Status"
  CSMA/CD/3(TxNext) -> Entity Input Switch1/2  "Admit Next Frame"
  Transmission Buffer/1 -> "Admit 1 Frame "/2
  "Admit 1 Frame "/1 -> "Merge "/2
  "Merge "/1 -> Wait for Channel/1
  Wait for Channel/1 -> Send to Channel/2
  Send to Channel/1 -> Copy Transmitted Frame/1
  Copy Transmitted Frame/2 -> CSMA/CD/1(TxIn)
  [rx2_1] -> CSMA/CD/2(RxIn)
  CSMA/CD/2(TxRe) -> "Merge "/1  "Retransmit Frame"
  Copy Transmitted Frame/1 -> [tx2_1]
  Assemble MAC Frame/1 -> Transmission Buffer/1
  DataIn/1 -> Copy Message/1
  Copy Message/2 -> Assemble MAC Frame/1
  Copy Message/1 -> Simulink Function/1(In)
  Entity Input Switch1/1 -> "Admit 1 Frame "/1
  Simulink Function3/1(Out) -> Entity Input Switch1/1

== system MsgEthernetMdl/Computer 3/Subsystem ==
  In1 : Inport
  Bus Creator : BusCreator  Inputs=4  OutDataTypeStr=Bus: dataPacket  NonVirtualBus=on
  Constant : Constant  Value=[10 1 1 3]
  Generate Data 1 : MATLAB Function  TreatAsAtomicUnit=on  SystemSampleTime=0.01
  Send : Send  OutputPortMessageModes=m
  out : Outport  InputPortMessageModes=m  OutDataTypeStr=Bus: dataPacket  BusOutputAsStruct=on
  wires:
  Constant/1 -> Bus Creator/2  "DestAddress"
  In1/1 -> Bus Creator/1  "SrcAddress"
  Send/1 -> out/1  "Message"
  Generate Data 1/2(PayloadSize) -> Bus Creator/4
  Bus Creator/1 -> Send/1
  Generate Data 1/1(Data) -> Bus Creator/3

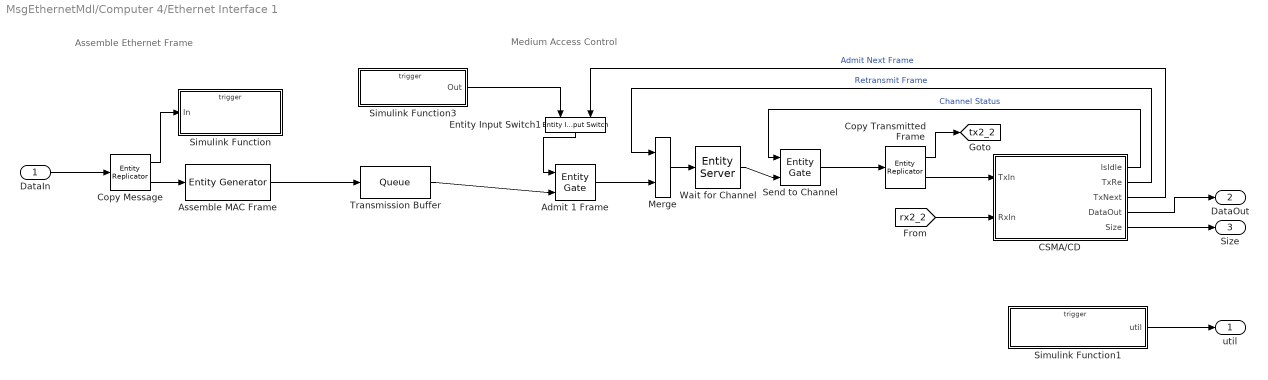
== system MsgEthernetMdl/Computer 4/Ethernet Interface 1 ==
  note: Assemble Ethernet Frame
  note: Medium Access Control
  DataIn : Inport
  "Admit 1 Frame " : EntityGate  InputPortMessageModes=m,m  OutputPortMessageModes=m  OpenGateAtSimulationStart=on
  Assemble MAC Frame : EntityGenerator  InputPortMessageModes=m  OutputPortMessageModes=m  GenerationMethod=Event-based  GenerateAction=|  EntityType=Bus object  EntityTypeName=ethernetPacket
      | entity.TxAddress = StationID;
      | [entity.Data, entity.RxAddress, entity.PayloadSize] = initPacket();
      | entity.TxDelay = (entity.PayloadSize+22)*8/BitRate;
      | entity.BackoffTime = 0;
      | entity.CRC = 0;
      settings: InputPortMap=u0
  CSMA/CD : Stateflow chart  TreatAsAtomicUnit=on
  Copy Message : EntityReplicator  InputPortMessageModes=m  OutputPortMessageModes=m,m
  Copy Transmitted Frame : EntityReplicator  InputPortMessageModes=m  OutputPortMessageModes=m,m
  Entity Input Switch1 : EntityInputSwitch  InputPortMessageModes=m,m  OutputPortMessageModes=m
  "Merge " : EntityInputSwitch  InputPortMessageModes=m,m  OutputPortMessageModes=m
  Send to Channel : EntityGate  InputPortMessageModes=m,m  OutputPortMessageModes=m  OpenGateAtSimulationStart=on
  Simulink Function : Subsystem  TreatAsAtomicUnit=on
  Simulink Function1 : Subsystem  TreatAsAtomicUnit=on
  Simulink Function3 : Subsystem  TreatAsAtomicUnit=on
  Transmission Buffer : Queue  InputPortMessageModes=m  OutputPortMessageModes=m  Capacity=TxBufferCapacity  ExitAction=gateControl();
  Wait for Channel : EntityServer  InputPortMessageModes=m  OutputPortMessageModes=m  Capacity=1  ServiceTimeSource=Attribute  ServiceTimeAttributeName=BackoffTime
  util : Outport
  DataOut : Outport  Port=2
  Size : Outport  Port=3
  tag scope: tx2_2=global
  wires:
  CSMA/CD/5(Size) -> Size/1
  Simulink Function1/1(util) -> util/1
  CSMA/CD/4(DataOut) -> DataOut/1
  CSMA/CD/1(IsIdle) -> Send to Channel/1  "Channel Status"
  CSMA/CD/3(TxNext) -> Entity Input Switch1/2  "Admit Next Frame"
  Transmission Buffer/1 -> "Admit 1 Frame "/2
  "Admit 1 Frame "/1 -> "Merge "/2
  "Merge "/1 -> Wait for Channel/1
  Wait for Channel/1 -> Send to Channel/2
  Send to Channel/1 -> Copy Transmitted Frame/1
  Copy Transmitted Frame/2 -> CSMA/CD/1(TxIn)
  [rx2_2] -> CSMA/CD/2(RxIn)
  CSMA/CD/2(TxRe) -> "Merge "/1  "Retransmit Frame"
  Copy Transmitted Frame/1 -> [tx2_2]
  Assemble MAC Frame/1 -> Transmission Buffer/1
  DataIn/1 -> Copy Message/1
  Copy Message/2 -> Assemble MAC Frame/1
  Copy Message/1 -> Simulink Function/1(In)
  Entity Input Switch1/1 -> "Admit 1 Frame "/1
  Simulink Function3/1(Out) -> Entity Input Switch1/1

== system MsgEthernetMdl/Computer 4/Subsystem ==
  In1 : Inport
  Bus Creator : BusCreator  Inputs=4  OutDataTypeStr=Bus: dataPacket  NonVirtualBus=on
  Constant : Constant  Value=[10 1 1 2]
  Generate Data 1 : MATLAB Function  TreatAsAtomicUnit=on  SystemSampleTime=0.01
  Send : Send  OutputPortMessageModes=m
  out : Outport  InputPortMessageModes=m  OutDataTypeStr=Bus: dataPacket  BusOutputAsStruct=on
  wires:
  Constant/1 -> Bus Creator/2  "DestAddress"
  In1/1 -> Bus Creator/1  "SrcAddress"
  Send/1 -> out/1  "Message"
  Generate Data 1/2(PayloadSize) -> Bus Creator/4
  Bus Creator/1 -> Send/1
  Generate Data 1/1(Data) -> Bus Creator/3

== system MsgEthernetMdl/Router1/Simulink Function ==
  Inport : Inport
  Inport1 : Inport  Port=2
  Inport2 : Inport  Port=3
  networkselector : TriggerPort  TriggerType=function-call  IsSimulinkFunction=on  FunctionName=networkselector  FunctionVisibility=scoped  VariantControl=(inherit)
  Bus Selector : BusSelector  OutputSignals=Data
  Bus Selector1 : BusSelector  OutputSignals=DestAddress
  MATLAB Function : MATLAB Function  TreatAsAtomicUnit=on
  Message Send : Send  OutputPortMessageModes=m
  Receive : Receive  InputPortMessageModes=m  UseInternalQueue=off  QueueOverwriting=on  QueueLength=1  QueueType=LIFO
  path : Outport
  wires:
  Receive/1 -> Bus Selector/1
  Inport/1 -> MATLAB Function/1(v1)
  Inport1/1 -> MATLAB Function/2(v2)
  Bus Selector/1 -> Bus Selector1/1  "<Data>"
  MATLAB Function/1(idx) -> Message Send/1
  Message Send/1 -> path/1
  Inport2/1 -> Receive/1
  Bus Selector1/1 -> MATLAB Function/3(dest)  "<DestAddress>"

== system MsgEthernetMdl/Router1/Simulink Function3 ==
  gateControl : TriggerPort  TriggerType=function-call  IsSimulinkFunction=on  FunctionName=gateControl  FunctionVisibility=scoped  VariantControl=Variant
  Constant : Constant  Value=0
  Message Send : Send  OutputPortMessageModes=m
  Out : Outport
  wires:
  Message Send/1 -> Out/1
  Constant/1 -> Message Send/1

== system MsgEthernetMdl/Computer 1/Ethernet Interface 1/Simulink Function ==
  In : Inport
  initPacket : TriggerPort  TriggerType=function-call  IsSimulinkFunction=on  FunctionName=initPacket  FunctionVisibility=scoped  VariantControl=(inherit)
  Bus Selector : BusSelector  OutputSignals=DestAddress,PayloadSize
  Constant : Constant
  Display : Display
  Receive : Receive  InputPortMessageModes=m  QueueLength=2^16-1
  Submatrix : matrix_library/Submatrix  RowSpan=Range of rows  RowStartMode=Last  RowStartIndex=1  RowEndMode=Last  RowEndIndex=1  ColSpan=Range of columns  ColStartMode=Last  ColStartIndex=1  ColEndMode=Last  ColEndIndex=1
      settings: SourceProductBaseCode=SL
  Subtract : Sum  Inputs=+-
  data : ArgOut  DisableCoverage=on  OutDataTypeStr=Bus: dataPacket  ArgumentName=data
  data2 : ArgOut  DisableCoverage=on  Port=2  ArgumentName=DestAddress
  data1 : ArgOut  DisableCoverage=on  Port=3  ArgumentName=payloadsize
  wires:
  In/1 -> Receive/1
  Receive/1 -> Bus Selector/1, data/1
  Bus Selector/2 -> data1/1  "<PayloadSize>"
  Bus Selector/1 -> Submatrix/1  "<DestAddress>"
  Submatrix/1 -> Subtract/1
  Constant/1 -> Subtract/2
  Subtract/1 -> Display/1, data2/1

== system MsgEthernetMdl/Computer 1/Ethernet Interface 1/Simulink Function1 ==
  compUtil : TriggerPort  TriggerType=function-call  IsSimulinkFunction=on  FunctionName=compUtil  FunctionVisibility=scoped  VariantControl=(inherit)
  Digital Clock : DigitalClock  SampleTime=-1
  MATLAB Function1 : MATLAB Function  TreatAsAtomicUnit=on
  isIdle : ArgIn  ArgumentName=isIdle
  util : Outport
  wires:
  Digital Clock/1 -> MATLAB Function1/1(t)
  isIdle/1 -> MATLAB Function1/2(isIdle)
  MATLAB Function1/1(util) -> util/1

== system MsgEthernetMdl/Computer 1/Ethernet Interface 1/Simulink Function3 ==
  gateControl : TriggerPort  TriggerType=function-call  IsSimulinkFunction=on  FunctionName=gateControl  FunctionVisibility=scoped  VariantControl=Variant
  Constant : Constant  Value=0
  Message Send : Send  OutputPortMessageModes=m
  Out : Outport
  wires:
  Message Send/1 -> Out/1
  Constant/1 -> Message Send/1

== system MsgEthernetMdl/Computer 2/Ethernet Interface 2/Simulink Function ==
  In : Inport
  initPacket : TriggerPort  TriggerType=function-call  IsSimulinkFunction=on  FunctionName=initPacket  FunctionVisibility=scoped  VariantControl=(inherit)
  Bus Selector : BusSelector  OutputSignals=DestAddress,PayloadSize
  Constant : Constant
  Display : Display
  Receive : Receive  InputPortMessageModes=m  QueueLength=2^16-1
  Submatrix : matrix_library/Submatrix  RowSpan=Range of rows  RowStartMode=Last  RowStartIndex=1  RowEndMode=Last  RowEndIndex=1  ColSpan=Range of columns  ColStartMode=Last  ColStartIndex=1  ColEndMode=Last  ColEndIndex=1
      settings: SourceProductBaseCode=SL
  Subtract : Sum  Inputs=+-
  data : ArgOut  DisableCoverage=on  OutDataTypeStr=Bus: dataPacket  ArgumentName=data
  data2 : ArgOut  DisableCoverage=on  Port=2  ArgumentName=DestAddress
  data1 : ArgOut  DisableCoverage=on  Port=3  ArgumentName=payloadsize
  wires:
  Constant/1 -> Subtract/2
  Subtract/1 -> Display/1, data2/1
  Bus Selector/1 -> Submatrix/1  "<DestAddress>"
  Submatrix/1 -> Subtract/1
  Receive/1 -> Bus Selector/1, data/1
  In/1 -> Receive/1
  Bus Selector/2 -> data1/1  "<PayloadSize>"

== system MsgEthernetMdl/Computer 2/Ethernet Interface 2/Simulink Function2 ==
  compUtil : TriggerPort  TriggerType=function-call  IsSimulinkFunction=on  FunctionName=compUtil  FunctionVisibility=scoped  VariantControl=(inherit)
  Digital Clock : DigitalClock  SampleTime=-1
  MATLAB Function1 : MATLAB Function  TreatAsAtomicUnit=on
  isIdle1 : ArgIn  ArgumentName=isIdle
  util : Outport
  wires:
  Digital Clock/1 -> MATLAB Function1/1(t)
  isIdle1/1 -> MATLAB Function1/2(isIdle)
  MATLAB Function1/1(util) -> util/1

== system MsgEthernetMdl/Computer 2/Ethernet Interface 2/Simulink Function3 ==
  gateControl : TriggerPort  TriggerType=function-call  IsSimulinkFunction=on  FunctionName=gateControl  FunctionVisibility=scoped  VariantControl=Variant
  Constant : Constant  Value=0
  Message Send : Send  OutputPortMessageModes=m
  Out : Outport
  wires:
  Message Send/1 -> Out/1
  Constant/1 -> Message Send/1

== system MsgEthernetMdl/Computer 3/Ethernet Interface 1/Simulink Function ==
  In : Inport
  initPacket : TriggerPort  TriggerType=function-call  IsSimulinkFunction=on  FunctionName=initPacket  FunctionVisibility=scoped  VariantControl=(inherit)
  Bus Selector : BusSelector  OutputSignals=DestAddress,PayloadSize
  Constant : Constant
  Display : Display
  Receive : Receive  InputPortMessageModes=m  QueueLength=2^16-1
  Submatrix : matrix_library/Submatrix  RowSpan=Range of rows  RowStartMode=Last  RowStartIndex=1  RowEndMode=Last  RowEndIndex=1  ColSpan=Range of columns  ColStartMode=Last  ColStartIndex=1  ColEndMode=Last  ColEndIndex=1
      settings: SourceProductBaseCode=SL
  Subtract : Sum  Inputs=+-
  data : ArgOut  DisableCoverage=on  OutDataTypeStr=Bus: dataPacket  ArgumentName=data
  data2 : ArgOut  DisableCoverage=on  Port=2  ArgumentName=DestAddress
  data1 : ArgOut  DisableCoverage=on  Port=3  ArgumentName=payloadsize
  wires:
  In/1 -> Receive/1
  Receive/1 -> Bus Selector/1, data/1
  Bus Selector/2 -> data1/1  "<PayloadSize>"
  Bus Selector/1 -> Submatrix/1  "<DestAddress>"
  Submatrix/1 -> Subtract/1
  Constant/1 -> Subtract/2
  Subtract/1 -> Display/1, data2/1

== system MsgEthernetMdl/Computer 3/Ethernet Interface 1/Simulink Function1 ==
  compUtil : TriggerPort  TriggerType=function-call  IsSimulinkFunction=on  FunctionName=compUtil  FunctionVisibility=scoped  VariantControl=(inherit)
  Digital Clock : DigitalClock  SampleTime=-1
  MATLAB Function1 : MATLAB Function  TreatAsAtomicUnit=on
  isIdle : ArgIn  ArgumentName=isIdle
  util : Outport
  wires:
  Digital Clock/1 -> MATLAB Function1/1(t)
  isIdle/1 -> MATLAB Function1/2(isIdle)
  MATLAB Function1/1(util) -> util/1

== system MsgEthernetMdl/Computer 3/Ethernet Interface 1/Simulink Function3 ==
  gateControl : TriggerPort  TriggerType=function-call  IsSimulinkFunction=on  FunctionName=gateControl  FunctionVisibility=scoped  VariantControl=Variant
  Constant : Constant  Value=0
  Message Send : Send  OutputPortMessageModes=m
  Out : Outport
  wires:
  Message Send/1 -> Out/1
  Constant/1 -> Message Send/1

== system MsgEthernetMdl/Computer 4/Ethernet Interface 1/Simulink Function ==
  In : Inport
  initPacket : TriggerPort  TriggerType=function-call  IsSimulinkFunction=on  FunctionName=initPacket  FunctionVisibility=scoped  VariantControl=(inherit)
  Bus Selector : BusSelector  OutputSignals=DestAddress,PayloadSize
  Constant : Constant
  Display : Display
  Receive : Receive  InputPortMessageModes=m  QueueLength=2^16-1
  Submatrix : matrix_library/Submatrix  RowSpan=Range of rows  RowStartMode=Last  RowStartIndex=1  RowEndMode=Last  RowEndIndex=1  ColSpan=Range of columns  ColStartMode=Last  ColStartIndex=1  ColEndMode=Last  ColEndIndex=1
      settings: SourceProductBaseCode=SL
  Subtract : Sum  Inputs=+-
  data : ArgOut  DisableCoverage=on  OutDataTypeStr=Bus: dataPacket  ArgumentName=data
  data2 : ArgOut  DisableCoverage=on  Port=2  ArgumentName=DestAddress
  data1 : ArgOut  DisableCoverage=on  Port=3  ArgumentName=payloadsize
  wires:
  In/1 -> Receive/1
  Receive/1 -> Bus Selector/1, data/1
  Bus Selector/2 -> data1/1  "<PayloadSize>"
  Bus Selector/1 -> Submatrix/1  "<DestAddress>"
  Submatrix/1 -> Subtract/1
  Constant/1 -> Subtract/2
  Subtract/1 -> Display/1, data2/1

== system MsgEthernetMdl/Computer 4/Ethernet Interface 1/Simulink Function1 ==
  compUtil : TriggerPort  TriggerType=function-call  IsSimulinkFunction=on  FunctionName=compUtil  FunctionVisibility=scoped  VariantControl=(inherit)
  Digital Clock : DigitalClock  SampleTime=-1
  MATLAB Function1 : MATLAB Function  TreatAsAtomicUnit=on
  isIdle : ArgIn  ArgumentName=isIdle
  util : Outport
  wires:
  Digital Clock/1 -> MATLAB Function1/1(t)
  isIdle/1 -> MATLAB Function1/2(isIdle)
  MATLAB Function1/1(util) -> util/1

== system MsgEthernetMdl/Computer 4/Ethernet Interface 1/Simulink Function3 ==
  gateControl : TriggerPort  TriggerType=function-call  IsSimulinkFunction=on  FunctionName=gateControl  FunctionVisibility=scoped  VariantControl=Variant
  Constant : Constant  Value=0
  Message Send : Send  OutputPortMessageModes=m
  Out : Outport
  wires:
  Message Send/1 -> Out/1
  Constant/1 -> Message Send/1

== matlab function MsgEthernetMdl/Computer 2/Ethernet Interface 2/Simulink Function2/MATLAB Function1 ==
  data: t input; util output; isIdle input
function util = fcn(t, isIdle)

persistent lastTime lastState totalUse;

if isempty(lastTime)
    lastTime = 0;
    lastState = 0;
    totalUse = 0;
end

if lastState ==1 % busy
    totalUse = totalUse + (t - lastTime);
end
lastTime = t;
if isIdle
    lastState = 0;
else
    lastState = 1;
end
if t > 0
    util = totalUse/t;
else
    util = lastState;
end
